simulink model "MIPS"  (R2017b)
settings: Solver=VariableStepAuto  StartTime=0.0  StopTime=20  RelTol=1e-3
libraries: xbsIndex_r4 x21
settings Model: Creator=manoh  LastModifiedBy=manoh

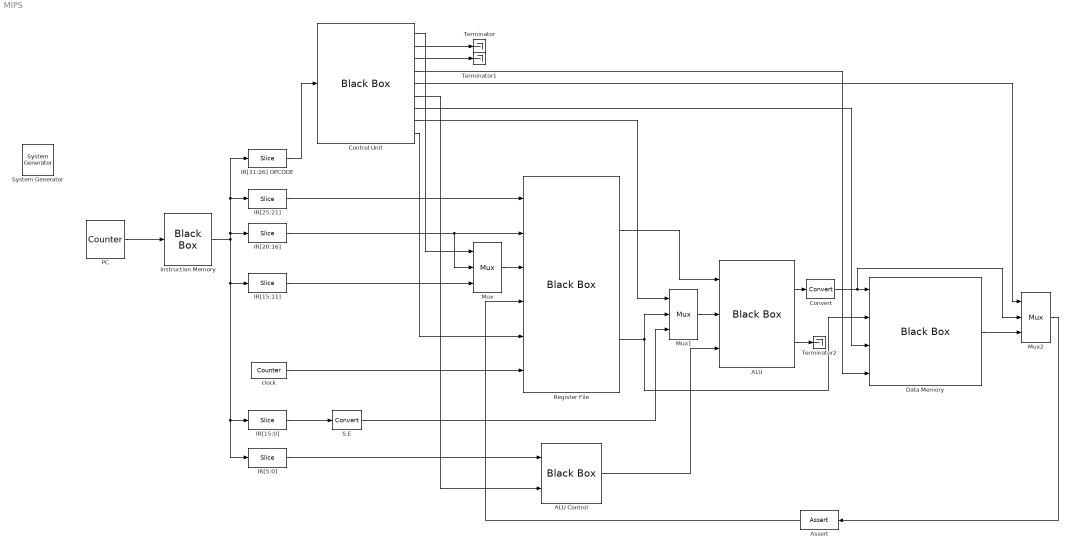
== system MIPS ==
  " System Generator" : xbsIndex_r4/ System Generator  Tag=genX  xilinxfamily=kintex7  part=xc7k325t  speed=-3  package=fbg676  synthesis_tool=Vivado  clock_wrapper=Clock Enables  directory=./netlist  proj_type=Vivado  Synth_file=Vivado Synthesis Defaults  Impl_file=Vivado Implementation Defaults  testbench=off  simulink_period=2  sysclk_period=10  dcm_input_clock_period=10  incr_netlist=off  trim_vbits=Everywhere in SubSystem  dbl_ovrd=According to Block Masks  core_generation=According to Block Masks  run_coregen=off  deprecated_control=off  eval_field=0  block_type=sysgen
  ALU : xbsIndex_r4/Black Box  init_code=ALU_config  sim_method=ISE Simulator  verbose=off  block_type=blackbox2
  ALU Control : xbsIndex_r4/Black Box  init_code=ALUControl_config  sim_method=ISE Simulator  verbose=off  block_type=blackbox2
  Assert : xbsIndex_r4/Assert  assert_type=on  type_source=Explicitly  gui_display_data_type=Fixed-point  arith_type="Signed  (2's comp)"  n_bits=32  bin_pt=0  preci_type=Single  exp_width=8  frac_width=24  assert_rate=off  rate_source=Explicitly  period=1  output_port=on  block_type=assert
  Control Unit : xbsIndex_r4/Black Box  init_code=ControlUnit_config  sim_method=ISE Simulator  verbose=off  block_type=blackbox2
  Convert : xbsIndex_r4/Convert  gui_display_data_type=Fixed-point  arith_type="Signed  (2's comp)"  n_bits=32  bin_pt=0  float_type=Single  exp_bits=8  fraction_bits=24  quantization=Truncate  overflow=Wrap  en=off  latency=1  pipeline=off  dbl_ovrd=off  block_type=convert
  Data Memory : xbsIndex_r4/Black Box  init_code=DataMemory_config  sim_method=ISE Simulator  verbose=off  block_type=blackbox2
  IR[15:0] : xbsIndex_r4/Slice  nbits=16  boolean_output=off  mode=Lower Bit Location + Width  bit1=-21  base1=MSB of Input  bit0=0  base0=LSB of Input  dbl_ovrd=off  block_type=slice
  IR[15:11] : xbsIndex_r4/Slice  nbits=5  boolean_output=off  mode=Upper Bit Location + Width  bit1=-16  base1=MSB of Input  bit0=0  base0=LSB of Input  dbl_ovrd=off  block_type=slice
  IR[20:16] : xbsIndex_r4/Slice  nbits=5  boolean_output=off  mode=Upper Bit Location + Width  bit1=-11  base1=MSB of Input  bit0=0  base0=LSB of Input  dbl_ovrd=off  block_type=slice
  IR[25:21] : xbsIndex_r4/Slice  nbits=5  boolean_output=off  mode=Upper Bit Location + Width  bit1=-6  base1=MSB of Input  bit0=0  base0=LSB of Input  dbl_ovrd=off  block_type=slice
  IR[31:26] OPCODE : xbsIndex_r4/Slice  nbits=6  boolean_output=off  mode=Upper Bit Location + Width  bit1=0  base1=MSB of Input  bit0=0  base0=LSB of Input  dbl_ovrd=off  block_type=slice
  IR[5:0] : xbsIndex_r4/Slice  nbits=6  boolean_output=off  mode=Lower Bit Location + Width  bit1=-16  base1=MSB of Input  bit0=0  base0=LSB of Input  dbl_ovrd=off  block_type=slice
  Instruction Memory : xbsIndex_r4/Black Box  init_code=InstructionMemory_config  sim_method=ISE Simulator  verbose=off  block_type=blackbox2
  Mux : xbsIndex_r4/Mux  inputs=2  en=off  latency=0  precision=Full  arith_type=Unsigned  n_bits=16  bin_pt=14  quantization=Truncate  overflow=Wrap  dbl_ovrd=off  block_type=mux
  Mux1 : xbsIndex_r4/Mux  inputs=2  en=off  latency=0  precision=User Defined  arith_type="Signed  (2's comp)"  n_bits=32  bin_pt=0  quantization=Truncate  overflow=Wrap  dbl_ovrd=off  block_type=mux
  Mux2 : xbsIndex_r4/Mux  inputs=2  en=off  latency=1  precision=User Defined  arith_type="Signed  (2's comp)"  n_bits=32  bin_pt=0  quantization=Truncate  overflow=Wrap  dbl_ovrd=off  block_type=mux
  PC : xbsIndex_r4/Counter  cnt_type=Free Running  cnt_to=Inf  operation=Up  start_count=0  cnt_by_val=4  arith_type=Unsigned  n_bits=32  bin_pt=0  load_pin=off  rst=off  en=off  explicit_period=on  period=2  use_behavioral_HDL=off  implementation=Fabric  dbl_ovrd=off  block_type=counter
  Register File : xbsIndex_r4/Black Box  init_code=regfile_config  sim_method=ISE Simulator  verbose=off  block_type=blackbox2
  S.E : xbsIndex_r4/Convert  gui_display_data_type=Fixed-point  arith_type="Signed  (2's comp)"  n_bits=32  bin_pt=0  float_type=Single  exp_bits=8  fraction_bits=24  quantization=Truncate  overflow=Wrap  en=off  latency=0  pipeline=off  dbl_ovrd=off  block_type=convert
  Terminator : Terminator
  Terminator1 : Terminator
  Terminator2 : Terminator
  clock : xbsIndex_r4/Counter  cnt_type=Free Running  cnt_to=Inf  operation=Up  start_count=0  cnt_by_val=1  arith_type=Unsigned  n_bits=1  bin_pt=0  load_pin=off  rst=off  en=off  explicit_period=on  period=2  use_behavioral_HDL=off  implementation=Fabric  dbl_ovrd=off  block_type=counter
  wires:
  PC/1 -> Instruction Memory/1
  Instruction Memory/1 -> IR[25:21]/1, IR[31:26] OPCODE/1, IR[20:16]/1, IR[5:0]/1, IR[15:0]/1, IR[15:11]/1
  IR[25:21]/1 -> Register File/1
  clock/1 -> Register File/6
  IR[31:26] OPCODE/1 -> Control Unit/1
  ALU Control/1 -> ALU/3
  Mux/1 -> Register File/3
  IR[20:16]/1 -> Mux/2, Register File/2
  IR[15:11]/1 -> Mux/3
  Control Unit/1 -> Mux/1
  Control Unit/9 -> Register File/5
  Mux1/1 -> ALU/2
  Register File/2 -> Data Memory/2, Mux1/2
  IR[15:0]/1 -> S.E/1
  S.E/1 -> Mux1/3
  IR[5:0]/1 -> ALU Control/1
  Control Unit/6 -> ALU Control/2
  Control Unit/8 -> Mux1/1
  ALU/1 -> Convert/1
  Control Unit/7 -> Data Memory/3
  Control Unit/4 -> Data Memory/4
  Control Unit/2 -> Terminator/1
  Control Unit/3 -> Terminator1/1
  ALU/2 -> Terminator2/1
  Mux2/1 -> Assert/1
  Register File/1 -> ALU/1
  Convert/1 -> Mux2/2, Data Memory/1
  Data Memory/1 -> Mux2/3
  Control Unit/5 -> Mux2/1
  Assert/1 -> Register File/4
